simulink model "ASMEqC"  (R2013b)
settings: Solver=ode45  StartTime=0.0  StopTime=10.0  RelTol=1e-3
undefined symbols (not defined in the file or in its folder): motor
libraries: fl_lib x9, nesl_utility x6, elec_lib x1
settings Model: Creator=sizuest  LastModifiedBy=sizuest

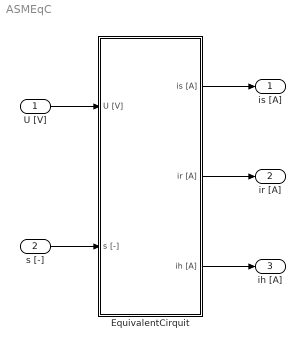
== system ASMEqC ==
  U [V] : Inport
  s [-] : Inport  Port=2
  EquivalentCirquit : Subsystem
  is [A] : Outport
  ir [A] : Outport  Port=2
  ih [A] : Outport  Port=3
  wires:
  U [V]/1 -> EquivalentCirquit/1(U [V])
  s [-]/1 -> EquivalentCirquit/2(s [-])
  EquivalentCirquit/1(is [A]) -> is [A]/1
  EquivalentCirquit/2(ir [A]) -> ir [A]/1
  EquivalentCirquit/3(ih [A]) -> ih [A]/1

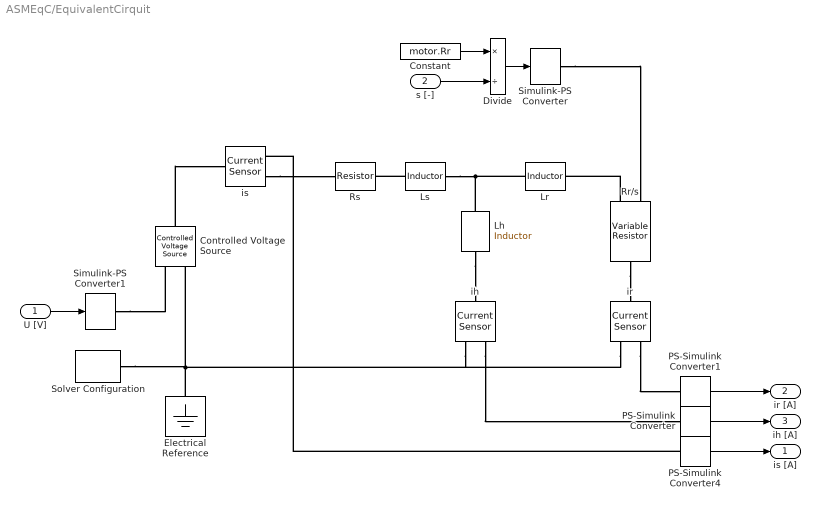
== system ASMEqC/EquivalentCirquit ==
  U [V] : Inport
  s [-] : Inport  Port=2
  Constant : Constant  Value=motor.Rr
  Controlled Voltage Source : fl_lib/Electrical/Electrical Sources/Controlled Voltage Source  i_Log=off  v_Log=off  LocalVarNames=|i|v  LocalVarDescs=|i|v  LocalVarLogging=[0 0]
  Divide : Product  Inputs=*/
  Electrical Reference : fl_lib/Electrical/Electrical Elements/Electrical Reference  i_Log=off  LocalVarNames=|i  LocalVarDescs=|i  LocalVarLogging=0
  Lh : fl_lib/Electrical/Electrical Elements/Inductor  l=motor.Lh H  i0=0 A  r=0 Ohm  g=1e-9 1/Ohm  i_Log=off  v_Log=off  i_L_Log=off  LocalVarNames=|i|v|i_L  LocalVarDescs=|i|v|Internal variable for current through inductor term  LocalVarLogging=[0 0 0]
  Lr : fl_lib/Electrical/Electrical Elements/Inductor  l=motor.Lr H  i0=0 A  r=0 Ohm  g=1e-9 1/Ohm  i_Log=off  v_Log=off  i_L_Log=off  LocalVarNames=|i|v|i_L  LocalVarDescs=|i|v|Internal variable for current through inductor term  LocalVarLogging=[0 0 0]
  Ls : fl_lib/Electrical/Electrical Elements/Inductor  l=motor.Ls H  i0=0 A  r=0 Ohm  g=1e-9 1/Ohm  i_Log=off  v_Log=off  i_L_Log=off  LocalVarNames=|i|v|i_L  LocalVarDescs=|i|v|Internal variable for current through inductor term  LocalVarLogging=[0 0 0]
  PS-Simulink Converter : nesl_utility/PS-Simulink Converter  PhysicalDomain=network_engine_domain  SubClassName=ps_output  LeftPortType=input  RightPortType=output  PseudoPeriodic=off  Frequencies=[]  Unit=1  AffineConversion=off
  PS-Simulink Converter1 : nesl_utility/PS-Simulink Converter  PhysicalDomain=network_engine_domain  SubClassName=ps_output  LeftPortType=input  RightPortType=output  PseudoPeriodic=off  Frequencies=[]  Unit=1  AffineConversion=off
  PS-Simulink Converter4 : nesl_utility/PS-Simulink Converter  PhysicalDomain=network_engine_domain  SubClassName=ps_output  LeftPortType=input  RightPortType=output  PseudoPeriodic=off  Frequencies=[]  Unit=1  AffineConversion=off
  Rr/s : fl_lib/Electrical/Electrical Elements/Variable Resistor  Rmin=0 Ohm  i_Log=off  v_Log=off  LocalVarNames=|i|v  LocalVarDescs=|i|v  LocalVarLogging=[0 0]
  Rs : elec_lib/Passive Devices/Resistor  R=motor.Rs Ohm  noise_mode=0  Tdevice=25 C  sample_time=0.001 s  repeatability=1  auto_seed=1811450916  user_seed=0  LocalVarLogging=[]
  Simulink-PS Converter : nesl_utility/Simulink-PS Converter  PhysicalDomain=network_engine_domain  SubClassName=ps_input  LeftPortType=input  RightPortType=output  PseudoPeriodic=off  Frequencies=[]  NoiseDistribution=none  NoiseParameters=[]  Unit=1  AffineConversion=off  InputFiltering=off  SimscapeFilterOrder=1  InputFilterTimeConstant=0.001  UdotUserProvided=1
  Simulink-PS Converter1 : nesl_utility/Simulink-PS Converter  PhysicalDomain=network_engine_domain  SubClassName=ps_input  LeftPortType=input  RightPortType=output  PseudoPeriodic=off  Frequencies=[]  NoiseDistribution=none  NoiseParameters=[]  Unit=1  AffineConversion=off  InputFiltering=off  SimscapeFilterOrder=1  InputFilterTimeConstant=0.001  UdotUserProvided=1
  Solver Configuration : nesl_utility/Solver Configuration  PhysicalDomain=network_engine_domain  SubClassName=solver  LeftPortType=input  RightPortType=generic  Accelerate=off  Tones=[]  Harmonics=[]  SimulateNoise=off  Profile=off  UseLocalSampling=off  EnableSwitchedLinearOptims=on  FrequencyDomain=off  UseCCode=off  RelTol=0.001  AbsTol=1e-06  MinStep=1e-09  ToWorkspace=off  DoDC=off  ResidualTolerance=1e-09  UseLocalSolver=off  LocalSolverChoice=NE_BACKWARD_EULER_ADVANCER  LocalSolverSampleTime=1/500000  DoFixedCost=off  MaxNonlinIter=3  MaxModeIter=2  LinearAlgebra=Full  DelaysMemoryBudget=1024
  ih : fl_lib/Electrical/Electrical Sensors/Current Sensor  i1_Log=off  v1_Log=off  LocalVarNames=|i1|v1  LocalVarDescs=|i1|v1  LocalVarLogging=[0 0]
  ir : fl_lib/Electrical/Electrical Sensors/Current Sensor  i1_Log=off  v1_Log=off  LocalVarNames=|i1|v1  LocalVarDescs=|i1|v1  LocalVarLogging=[0 0]
  is : fl_lib/Electrical/Electrical Sensors/Current Sensor  i1_Log=off  v1_Log=off  LocalVarNames=|i1|v1  LocalVarDescs=|i1|v1  LocalVarLogging=[0 0]
  is [A] : Outport
  ir [A] : Outport  Port=2
  ih [A] : Outport  Port=3
  wires:
  PS-Simulink Converter/1 -> ih [A]/1
  s [-]/1 -> Divide/2
  U [V]/1 -> Simulink-PS Converter1/1
  Divide/1 -> Simulink-PS Converter/1
  PS-Simulink Converter1/1 -> ir [A]/1
  PS-Simulink Converter4/1 -> is [A]/1
  Constant/1 -> Divide/1
  connections:
  Lh/RConn1 -- ih/LConn1
  is/RConn2 -- Rs/LConn1
  Electrical Reference/LConn1 -- ir/RConn2 -- ih/RConn2 -- Solver Configuration/RConn1 -- Controlled Voltage Source/RConn2
  Rr/s/RConn1 -- ir/LConn1
  ih/RConn1 -- PS-Simulink Converter/LConn1
  Simulink-PS Converter/RConn1 -- Rr/s/LConn1
  Simulink-PS Converter1/RConn1 -- Controlled Voltage Source/RConn1
  Controlled Voltage Source/LConn1 -- is/LConn1
  ir/RConn1 -- PS-Simulink Converter1/LConn1
  PS-Simulink Converter4/LConn1 -- is/RConn1
  Lr/LConn1 -- Lh/LConn1 -- Ls/RConn1
  Ls/LConn1 -- Rs/RConn1
  Rr/s/LConn2 -- Lr/RConn1
